simulink model "simulacion_controlador_lqr_con_observador"  (R2015a)
settings: Solver=ode45  StartTime=0.0  StopTime=180  RelTol=1e-3
values from neighbouring files (symbols this model uses):
  g = 9.81    [bola_viga_con_obs.m]    (also in bola_viga_entrada_vel.m)
  Ib = 0.4*m*R^2    (= 4.624e-05)    [bola_viga_con_obs.m]    (also in bola_viga_entrada_vel.m)
  Iv = (Mb*(L)^2)/12    (= 0.0833333333333)    [bola_viga_con_obs.m]    (also in bola_viga_entrada_vel.m)
  L1 = place(AD',(CD*AD)',Pzo)'    [bola_viga_con_obs.m]    (also in bola_viga_entrada_vel.m)
  m = 0.1    [bola_viga_con_obs.m]    (also in bola_viga_entrada_vel.m)
  R = 0.034    [bola_viga_con_obs.m]    (also in bola_viga_entrada_vel.m)
  T = 0.06    [bola_viga_con_obs.m]    (also in bola_viga_entrada_vel.m)
undefined symbols (not defined in the file or in its folder): AD, BD, CD, K1
libraries: simulink x2
settings Model: Creator=HAROLD  LastModifiedBy=HAROLD

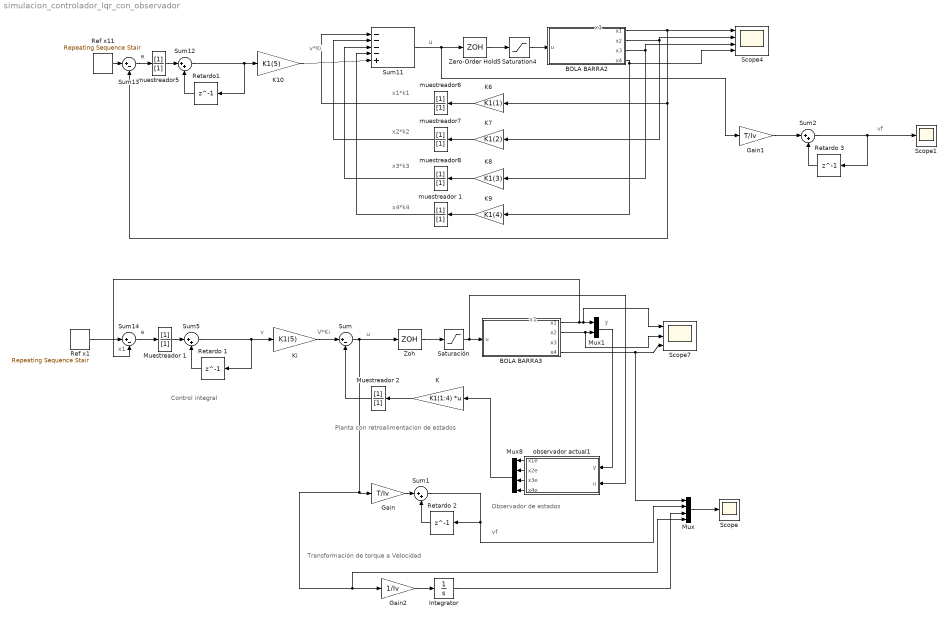
== system simulacion_controlador_lqr_con_observador ==
  note: x1
  note: V*Ki
  note: x4*k4
  note: x3*k3
  note: x2*k2
  note: x1*k1
  note: u
  note: v*Ki
  note: e
  note: x1
  note: y
  note: u
  note: v
  note: e
  note: x1
  note: Planta con retroalimentacion de estados
  note: Control integral
  note: Observador de estados
  note: vf
  note: vf
  note: Transformación de torque a Velocidad
  BOLA BARRA2 : Subsystem
  BOLA BARRA3 : Subsystem
  Gain : Gain  Gain=T/Iv
  Gain1 : Gain  Gain=T/Iv
  Gain2 : Gain  Gain=1/Iv
  Integrator : Integrator
  K : Gain  Gain=K1(1:4)  Multiplication=Matrix(K*u)
  K10 : Gain  Gain=K1(5)
  K6 : Gain  Gain=K1(1)
  K7 : Gain  Gain=K1(2)
  K8 : Gain  Gain=K1(3)
  K9 : Gain  Gain=K1(4)
  Ki : Gain  Gain=K1(5)
  Muestreador 1 : DiscreteFilter  Denominator=[1]  SampleTime=T
  Muestreador 2 : DiscreteFilter  Denominator=[1]  SampleTime=T
  Mux : Mux
  Mux1 : Mux  Inputs=2
  Mux8 : Mux
  Ref x1 : simulink/Sources/Repeating Sequence Stair  OutValues="[0.2  0.4 -0.4 -0.1 -0.3].'"  tsamp=36  OutMin=[]  OutMax=[]  OutDataTypeStr=double  OutputDataTypeScalingMode=double  OutDataType=fixdt(0,8)  ConRadixGroup=Best Precision: Vector-wise  OutScaling=2^-12
  Ref x11 : simulink/Sources/Repeating Sequence Stair  OutValues="[0.2  0.4 -0.4 -0.1 -0.3].'"  tsamp=36  OutMin=[]  OutMax=[]  OutDataTypeStr=double  OutputDataTypeScalingMode=double  OutDataType=fixdt(0,8)  ConRadixGroup=Best Precision: Vector-wise  OutScaling=2^-12
  Retardo 1 : Delay  DelayLength=1  SampleTime=T
  Retardo 2 : Delay  DelayLength=1  InitialCondition=0  SampleTime=T
  Retardo 3 : Delay  DelayLength=1  InitialCondition=0  SampleTime=T
  Retardo1 : Delay  DelayLength=1  SampleTime=T
  Saturación : Saturate  UpperLimit=2.11  LowerLimit=-2.11
  Saturation4 : Saturate  UpperLimit=2.11  LowerLimit=-2.11
  Scope : Scope
      settings: TimeRange=16  YMin=11.15191986644406  YMax=51.15191986644406
  Scope1 : Scope
  Scope4 : Scope  NumInputPorts=4
      settings: YMin=-5~-5~-5~-5  YMax=5~5~5~5  SaveName=datos
  Scope7 : Scope  NumInputPorts=3
      settings: YMin=-5~-5~-5  YMax=5~5~5  SaveName=datos1
  Sum : Sum  Inputs=|+-
  Sum{1..2,5,12} (4 alike) : Sum  Inputs=|++
  Sum11 : Sum  Inputs=|----+
  Sum13 : Sum  Inputs=|+-
  Sum14 : Sum  Inputs=|+-
  Zero-Order Hold5 : ZeroOrderHold  SampleTime=T
  Zoh : ZeroOrderHold  SampleTime=T
  muestreador 1 : DiscreteFilter  Denominator=[1]  SampleTime=T
  muestreador{5..8} (4 alike) : DiscreteFilter  Denominator=[1]  SampleTime=T
  observador actual1 : Subsystem
  wires:
  Sum11/1 -> Gain1/1, Zero-Order Hold5/1
  K6/1 -> muestreador6/1
  K7/1 -> muestreador7/1
  K8/1 -> muestreador8/1
  K9/1 -> muestreador 1/1
  Zero-Order Hold5/1 -> Saturation4/1
  muestreador6/1 -> Sum11/1
  muestreador7/1 -> Sum11/2
  muestreador8/1 -> Sum11/3
  muestreador 1/1 -> Sum11/4
  Sum13/1 -> muestreador5/1
  Retardo1/1 -> Sum12/2
  Sum12/1 -> Retardo1/1, K10/1
  K10/1 -> Sum11/5
  BOLA BARRA2/1(x1) -> Scope4/1, Sum13/2, K6/1
  muestreador5/1 -> Sum12/1
  Ref x11/1 -> Sum13/1
  Saturation4/1 -> BOLA BARRA2/1(u)
  BOLA BARRA2/2(x2) -> K7/1, Scope4/2
  BOLA BARRA2/3(x3) -> K8/1, Scope4/3
  BOLA BARRA2/4(x4) -> Scope4/4, K9/1
  K/1 -> Muestreador 2/1
  Zoh/1 -> Saturación/1
  Sum14/1 -> Muestreador 1/1
  Retardo 1/1 -> Sum5/2
  Sum5/1 -> Retardo 1/1, Ki/1
  Ki/1 -> Sum/1
  Muestreador 1/1 -> Sum5/1
  Ref x1/1 -> Sum14/1
  Muestreador 2/1 -> Sum/2
  BOLA BARRA3/1(x1) -> Sum14/2, Scope7/1, Mux1/1
  Saturación/1 -> observador actual1/2(u), BOLA BARRA3/1(u)
  observador actual1/1(x1e) -> Mux8/1
  observador actual1/2(x2e) -> Mux8/2
  observador actual1/3(x3e) -> Mux8/3
  observador actual1/4(x4e) -> Mux8/4
  Mux8/1 -> K/1
  BOLA BARRA3/2(x2) -> Scope7/2, Mux1/2
  Mux1/1 -> observador actual1/1(y)
  Sum/1 -> Mux/4, Gain2/1, Gain/1, Zoh/1
  Sum1/1 -> Mux/2, Retardo 2/1
  BOLA BARRA3/4(x4) -> Mux/1, Scope7/3
  Mux/1 -> Scope/1
  Retardo 2/1 -> Sum1/2
  Gain/1 -> Sum1/1
  Sum2/1 -> Scope1/1, Retardo 3/1
  Retardo 3/1 -> Sum2/2
  Gain1/1 -> Sum2/1
  Gain2/1 -> Integrator/1
  Integrator/1 -> Mux/3

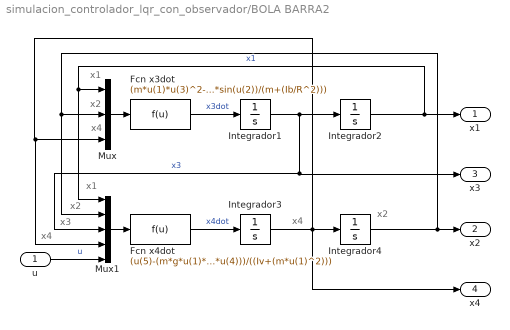
== system simulacion_controlador_lqr_con_observador/BOLA BARRA2 ==
  note: x4
  note: x3
  note: x2
  note: x1
  note: x4
  note: x2
  note: x1
  note: x2
  note: x4
  u : Inport
  Fcn x3dot : Fcn  Expr=(m*u(1)*u(3)^2-m*g*sin(u(2))/(m+(Ib/R^2)))
  Fcn x4dot : Fcn  Expr=(u(5)-(m*g*u(1)*cos(u(2)))-(2*m*u(1)*u(3)*u(4)))/((Iv+(m*u(1)^2)))
  Integrador1 : Integrator
  Integrador2 : Integrator  InitialCondition=-10.2e-3
  Integrador3 : Integrator
  Integrador4 : Integrator
  Mux : Mux  Inputs=3
  Mux1 : Mux  Inputs=5
  x1 : Outport
  x2 : Outport  Port=2
  x3 : Outport  Port=3
  x4 : Outport  Port=4
  wires:
  Mux1/1 -> Fcn x4dot/1
  Integrador2/1 -> Mux1/1, Mux/1, x1/1  "x1"
  Mux/1 -> Fcn x3dot/1
  Integrador1/1 -> Mux1/3, x3/1, Integrador2/1  "x3"
  Integrador3/1 -> x4/1, Mux1/4, Mux/3, Integrador4/1
  Integrador4/1 -> Mux1/2, Mux/2, x2/1
  Fcn x3dot/1 -> Integrador1/1  "x3dot"
  Fcn x4dot/1 -> Integrador3/1  "x4dot"
  u/1 -> Mux1/5  "u"

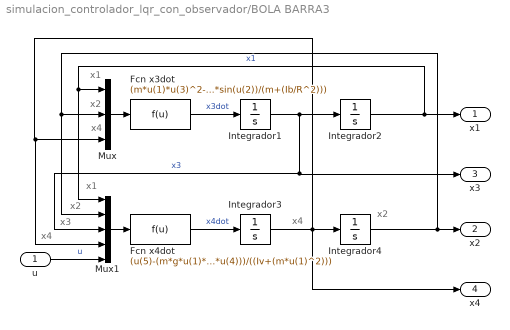
== system simulacion_controlador_lqr_con_observador/BOLA BARRA3 ==
  note: x4
  note: x3
  note: x2
  note: x1
  note: x4
  note: x2
  note: x1
  note: x2
  note: x4
  u : Inport
  Fcn x3dot : Fcn  Expr=(m*u(1)*u(3)^2-m*g*sin(u(2))/(m+(Ib/R^2)))
  Fcn x4dot : Fcn  Expr=(u(5)-(m*g*u(1)*cos(u(2)))-(2*m*u(1)*u(3)*u(4)))/((Iv+(m*u(1)^2)))
  Integrador1 : Integrator
  Integrador2 : Integrator  InitialCondition=-10.2e-3
  Integrador3 : Integrator
  Integrador4 : Integrator
  Mux : Mux  Inputs=3
  Mux1 : Mux  Inputs=5
  x1 : Outport
  x2 : Outport  Port=2
  x3 : Outport  Port=3
  x4 : Outport  Port=4
  wires:
  Mux1/1 -> Fcn x4dot/1
  Integrador2/1 -> Mux1/1, Mux/1, x1/1  "x1"
  Mux/1 -> Fcn x3dot/1
  Integrador1/1 -> Mux1/3, x3/1, Integrador2/1  "x3"
  Integrador3/1 -> x4/1, Mux1/4, Mux/3, Integrador4/1
  Integrador4/1 -> Mux1/2, Mux/2, x2/1
  Fcn x3dot/1 -> Integrador1/1  "x3dot"
  Fcn x4dot/1 -> Integrador3/1  "x4dot"
  u/1 -> Mux1/5  "u"

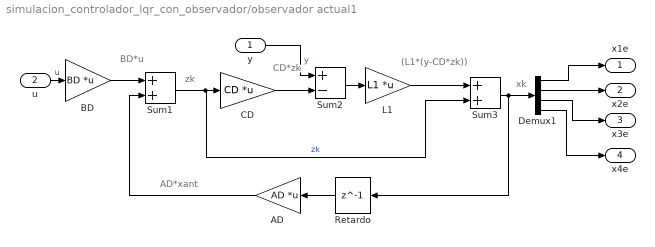
== system simulacion_controlador_lqr_con_observador/observador actual1 ==
  note: xk
  note: (L1*(y-CD*zk))
  note: CD*zk
  note: AD*xant
  note: BD*u
  note: zk
  y : Inport
  u : Inport  Port=2
  AD : Gain  Gain=AD  Multiplication=Matrix(K*u)
  BD : Gain  Gain=BD  Multiplication=Matrix(K*u)
  CD : Gain  Gain=CD  Multiplication=Matrix(K*u)
  Demux1 : Demux
  L1 : Gain  Gain=L1  Multiplication=Matrix(K*u)
  Retardo : Delay  DelayLength=1  InitialCondition=[0 0 0 0]  SampleTime=T
  Sum1 : Sum
  Sum2 : Sum  Inputs=+-
  Sum3 : Sum
  x1e : Outport
  x2e : Outport  Port=2
  x3e : Outport  Port=3
  x4e : Outport  Port=4
  wires:
  Demux1/1 -> x1e/1
  Demux1/2 -> x2e/1
  Demux1/3 -> x3e/1
  Demux1/4 -> x4e/1
  Sum2/1 -> L1/1
  Sum1/1 -> Sum3/2, CD/1  "zk"
  Sum3/1 -> Demux1/1, Retardo/1
  BD/1 -> Sum1/1
  AD/1 -> Sum1/2
  L1/1 -> Sum3/1
  CD/1 -> Sum2/2
  Retardo/1 -> AD/1
  u/1 -> BD/1  "u"
  y/1 -> Sum2/1  "y"
